simulink model "matlab_ppg_v1"  (R2018a)
settings: Solver=FixedStepAuto  StartTime=0.0  StopTime=inf  RelTol=1e-3  EnableMultiTasking=on
libraries: dspstat3 x8, dsparch4 x5, arduinolib x1, dspsrcs4 x1, neural x1
settings Model: SimulationMode=external  ExtModeTrigDuration=2  Creator=Na-Teng  LastModifiedBy=Na-Teng
settings SolverCC: AutoInsertRateTranBlk=on
settings OptimizationCC: EnhancedBackFolding=on  PassReuseOutputArgsAs=Individual arguments  MaxStackSize=64  OptimizeBlockOrder=speed  DifferentSizesBufferReuse=on  OptimizationCustomize=off
settings DebuggingCC: ParameterTunabilityLossMsg=error
settings HardwareCC: ProdBitPerInt=16  ProdBitPerPointer=16  ProdBitPerSizeT=16  ProdBitPerPtrDiffT=16  ProdLargestAtomicFloat=None  ProdWordSize=8  ProdHWDeviceType=Atmel->AVR
settings SFSimCC: MATLABDynamicMemAlloc=off
settings RTWCC: SystemTargetFile=ert.tlc  HardwareBoard=Arduino Mega 2560  TLCOptions=-aInlineSetEventsForThisBaseRateFcn=TLC_FALSE -aSuppressMultiTaskScheduler=TLC_FALSE -aRateBasedStepFcn=1  TemplateMakefile=ert_default_tmf  GenerateReport=on  Toolchain=Arduino AVR  BuildConfiguration=Faster Runs  IncludeHyperlinkInReport=on  LaunchReport=on  GenerateTraceInfo=on  GenerateTraceReport=on  GenerateTraceReportSl=on  GenerateTraceReportSf=on  GenerateTraceReportEml=on
settings CodeAppCC: ForceParamTrailComments=on  IgnoreCustomStorageClasses=off  OperatorAnnotations=on  SimulinkDataObjDesc=on  SFDataObjDesc=on  InsertBlockDesc=on
settings ERTTargetCC: SupportContinuousTime=on  SupportVariableSizeSignals=on

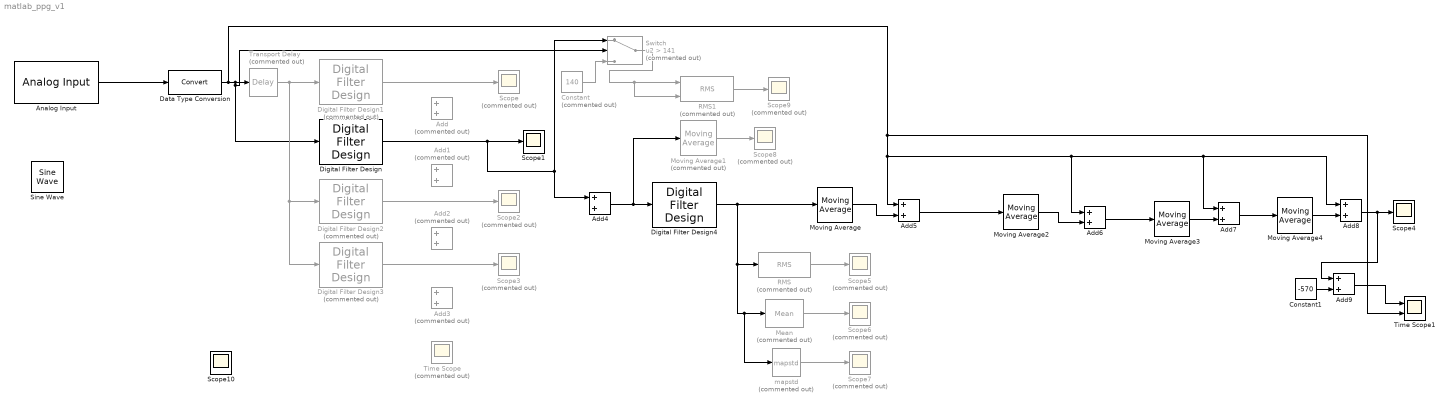
== system matlab_ppg_v1 ==
  Add{,1..3} (4 alike) : Sum  Commented=on
  Add{4..9} (6 alike) : Sum
  Analog Input : arduinolib/Analog Input  pinNumber=4  ReadResultsOnly=off  ConversionTriggerSource=Software  ExternalTriggerType=uint32(0)  OutputDataType=uint16  EnableConversionCompleteNotify=off  EnableOuputStatus=off  SampleTime=0.001  blockPlatform=arduino
  Constant : Constant  Commented=on  Value=140
  Constant1 : Constant  Value=-570
  Data Type Conversion : DataTypeConversion
  Digital Filter Design : dsparch4/Digital Filter Design  mwdsp_browser_bugfix_var=off
  Digital Filter Design1 : dsparch4/Digital Filter Design  Commented=on  mwdsp_browser_bugfix_var=off
  Digital Filter Design2 : dsparch4/Digital Filter Design  Commented=on  mwdsp_browser_bugfix_var=off
  Digital Filter Design3 : dsparch4/Digital Filter Design  Commented=on  mwdsp_browser_bugfix_var=off
  Digital Filter Design4 : dsparch4/Digital Filter Design  mwdsp_browser_bugfix_var=off
  Mean : dspstat3/Mean  Commented=on  run=off  InputProcessing=Columns as channels (frame based)  reset_popup=None  directionMode=Each column  dimension=1  roiEnable=off  roiType=Rectangles  roiPortion=Entire ROI  roiOutput=Individual statistics for each ROI  roiFlag=off  roundingMode=Floor  overflowMode=off  outputDataTypeStr=Inherit: Same as accumulator  outputMin=[]  outputMax=[]  outputLastDataTypeStr=Inherit: Same as accumulator
  Moving Average{,2..4} (4 alike) : dspstat3/Moving Average  Method=Exponential weighting  ForgettingFactorPort=off  SpecifyWindowLength=on  WindowLength=1  ForgettingFactor=0.9  SimulateUsing=Code generation
  Moving Average1 : dspstat3/Moving Average  Commented=on  Method=Sliding window  ForgettingFactorPort=off  SpecifyWindowLength=on  WindowLength=1  ForgettingFactor=0.9  SimulateUsing=Code generation
  RMS : dspstat3/RMS  Commented=on  run=off  directionMode=Each column  dimension=1  reset_popup=None
  RMS1 : dspstat3/RMS  Commented=on  run=on  directionMode=Each column  dimension=1  reset_popup=Falling edge
  Scope{,2..3,5..9} (8 alike) : Scope  Commented=on
  Scope1 : Scope
  Scope10 : Scope
  Scope4 : Scope
  Sine Wave : dspsrcs4/Sine Wave  Amplitude=1  Frequency=100  Phase=0  SampleMode=Continuous  OutComplex=Real  CompMethod=Trigonometric fcn  TableSize=Speed  SampleTime=0.001  SamplesPerFrame=1  ResetState=Restart at time zero  OutputFrames=off  dataType=double  wordLen=16  udDataType=sfix(16)  fracBitsMode=Best precision  numFracBits=15  OutDataTypeStr=double  LastOutDataTypeStr=double
  Switch : Switch  Commented=on  Criteria=u2 > Threshold  Threshold=141
  Time Scope : Scope  Commented=on  NumInputPorts=3
  Time Scope1 : Scope  NumInputPorts=2
  Transport Delay : TransportDelay  Commented=on  DelayTime=2
  mapstd : neural/Processing Functions/mapstd  Commented=on  xmean=500  xstd=[1; 1; 2]  ymean=-1  ystd=+1
      settings: SourceProductName=Neural Network Toolbox  SourceProductBaseCode=NN
  wires:
  Digital Filter Design1/1 -> Scope/1
  Digital Filter Design2/1 -> Scope2/1
  Digital Filter Design3/1 -> Scope3/1
  Data Type Conversion/1 -> Time Scope1/2, Add8/1, Add7/1, Add6/1, Add5/1, Switch/2, Digital Filter Design/1, Transport Delay/1
  Digital Filter Design4/1 -> mapstd/1, Mean/1, RMS/1, Moving Average/1
  mapstd/1 -> Scope7/1
  Mean/1 -> Scope6/1
  RMS/1 -> Scope5/1
  Moving Average1/1 -> Scope8/1
  Add4/1 -> Moving Average1/1, Digital Filter Design4/1
  Digital Filter Design/1 -> Switch/1, Add4/1, Scope1/1
  RMS1/1 -> Scope9/1
  Transport Delay/1 -> Digital Filter Design3/1, Digital Filter Design2/1, Digital Filter Design1/1
  Constant/1 -> Switch/3
  Switch/1 -> RMS1/2, RMS1/1
  Add5/1 -> Moving Average2/1
  Add6/1 -> Moving Average3/1
  Moving Average3/1 -> Add7/2
  Moving Average4/1 -> Add8/2
  Analog Input/1 -> Data Type Conversion/1
  Add7/1 -> Moving Average4/1
  Add8/1 -> Add9/1, Scope4/1
  Moving Average/1 -> Add5/2
  Moving Average2/1 -> Add6/2
  Constant1/1 -> Add9/2
  Add9/1 -> Time Scope1/1
